simulink model "Dynamic_model_2021a"  (R2021a)
settings: Solver=VariableStepAuto  StartTime=0.0  StopTime=10.0  RelTol=1e-3
libraries: dspmtrx3 x1, sharedtransform x1
settings Model: Creator=volko  LastModifiedBy=volko

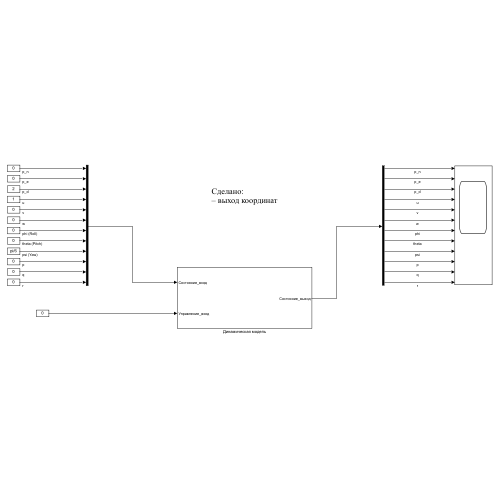
[thumbnail: Simulink's stored preview of the top-level diagram]
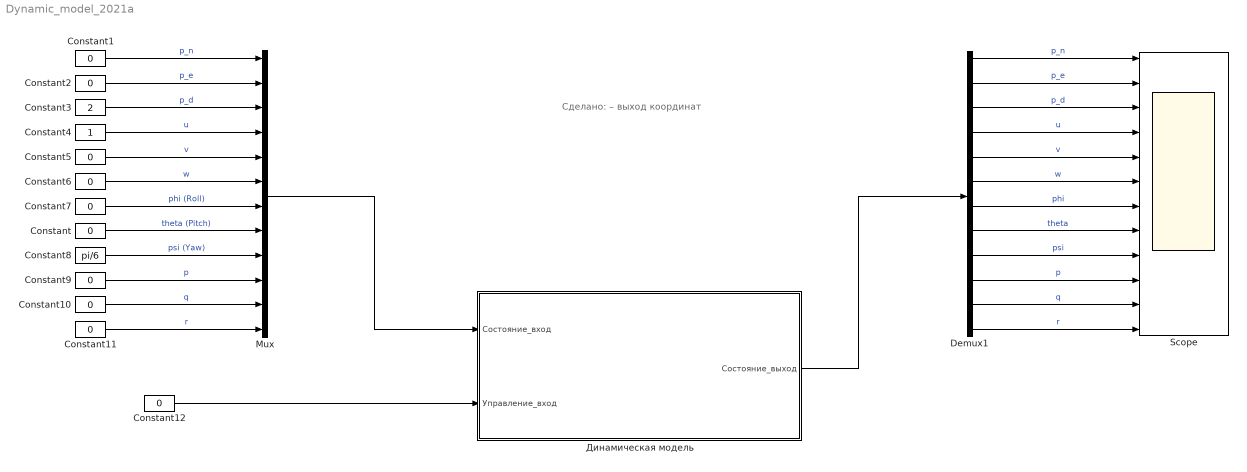
== system Dynamic_model_2021a ==
  note: Сделано:
      | – выход координат
  Constant{,1..2,5..7,9..12} (10 alike) : Constant  Value=0
  Constant3 : Constant  Value=2
  Constant4 : Constant
  Constant8 : Constant  Value=pi/6
  Demux1 : Demux  Outputs=12
  Mux : Mux  Inputs=12
  Scope : Scope  NumInputPorts=12
  Динамическая модель : Subsystem
  wires:
  Constant/1 -> Mux/8  "theta (Pitch)"
  Constant1/1 -> Mux/1  "p_n"
  Constant2/1 -> Mux/2  "p_e"
  Constant3/1 -> Mux/3  "p_d"
  Constant6/1 -> Mux/6  "w"
  Constant5/1 -> Mux/5  "v"
  Constant7/1 -> Mux/7  "phi (Roll)"
  Constant9/1 -> Mux/10  "p"
  Constant8/1 -> Mux/9  "psi (Yaw)"
  Constant10/1 -> Mux/11  "q"
  Constant11/1 -> Mux/12  "r"
  Mux/1 -> Динамическая модель/1(Состояние_вход)
  Constant12/1 -> Динамическая модель/2(Управление_вход)
  Динамическая модель/1(Состояние_выход) -> Demux1/1
  Demux1/1 -> Scope/1  "p_n"
  Demux1/2 -> Scope/2  "p_e"
  Demux1/3 -> Scope/3  "p_d"
  Constant4/1 -> Mux/4  "u"
  Demux1/4 -> Scope/4  "u"
  Demux1/5 -> Scope/5  "v"
  Demux1/6 -> Scope/6  "w"
  Demux1/7 -> Scope/7  "phi"
  Demux1/8 -> Scope/8  "theta"
  Demux1/9 -> Scope/9  "psi"
  Demux1/10 -> Scope/10  "p"
  Demux1/11 -> Scope/11  "q"
  Demux1/12 -> Scope/12  "r"

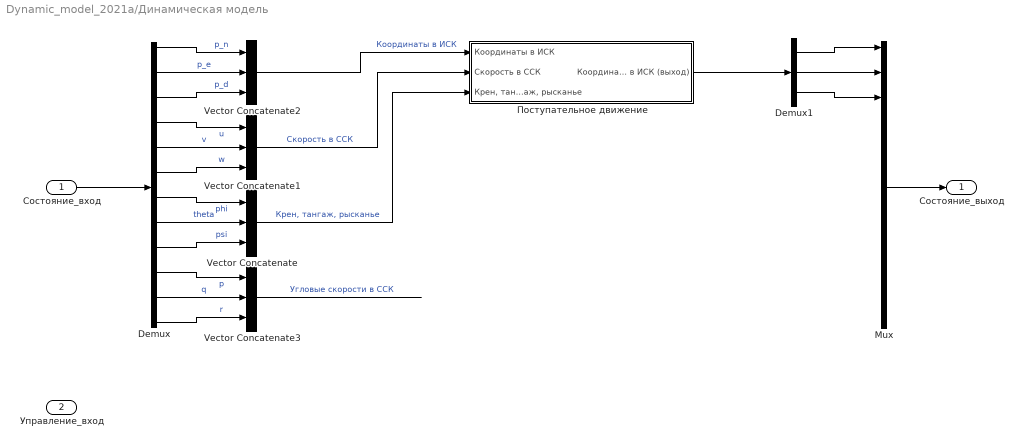
== system Dynamic_model_2021a/Динамическая модель ==
  Состояние_вход : Inport
  Управление_вход : Inport  Port=2
  Demux : Demux  Outputs=12
  Demux1 : Demux  Outputs=3
  Mux : Mux  Inputs=12
  Vector Concatenate{,1..3} (4 alike) : Concatenate  NumInputs=3
  Поступательное движение : Subsystem
  Состояние_выход : Outport
  wires:
  Состояние_вход/1 -> Demux/1
  Demux/1 -> Vector Concatenate2/1  "p_n"
  Demux/2 -> Vector Concatenate2/2  "p_e"
  Demux/3 -> Vector Concatenate2/3  "p_d"
  Demux/4 -> Vector Concatenate1/1  "u"
  Demux/5 -> Vector Concatenate1/2  "v"
  Demux/6 -> Vector Concatenate1/3  "w"
  Demux/7 -> Vector Concatenate/1  "phi"
  Demux/8 -> Vector Concatenate/2  "theta"
  Demux/9 -> Vector Concatenate/3  "psi"
  Demux/10 -> Vector Concatenate3/1  "p"
  Demux/11 -> Vector Concatenate3/2  "q"
  Demux/12 -> Vector Concatenate3/3  "r"
  Vector Concatenate2/1 -> Поступательное движение/1(Координаты в ИСК)  "Координаты в ИСК"
  Vector Concatenate1/1 -> Поступательное движение/2(Скорость в ССК)  "Скорость в ССК"
  Vector Concatenate/1 -> Поступательное движение/3("Крен, тангаж, рысканье")  "Крен, тангаж, рысканье"
  Поступательное движение/1(Координаты в ИСК (выход)) -> Demux1/1
  Vector Concatenate3/1 -> ?  "Угловые скорости в ССК"
  Mux/1 -> Состояние_выход/1
  Demux1/1 -> Mux/1
  Demux1/2 -> Mux/2
  Demux1/3 -> Mux/3

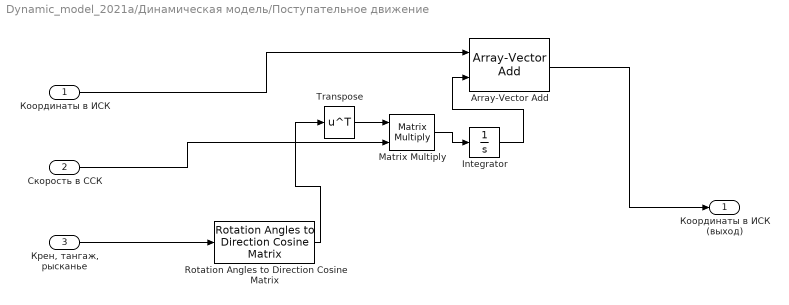
== system Dynamic_model_2021a/Динамическая модель/Поступательное движение ==
  Координаты в ИСК : Inport
  Скорость в ССК : Inport  Port=2
  "Крен, тангаж, рысканье" : Inport  Port=3
  Array-Vector Add : dspmtrx3/Array-Vector Add  Dimension=1  V_Source=Input port  V_VectFromMask=[0.5 0.25]  prodOutputSignedness=Auto  roundingMode=Floor  overflowMode=off  firstCoeffSignedness=Auto  firstCoeffDataTypeStr=Inherit: Same word length as input  firstCoeffMin=[]  firstCoeffMax=[]  firstCoeffLastDataTypeStr=Inherit: Same word length as input  accumSignedness=Auto  outputSignedness=Auto  outputDataTypeStr=Inherit: Same as accumulator  outputMin=[]  outputMax=[]  outputLastDataTypeStr=Inherit: Same as accumulator
      settings: SourceProductBaseCode=DS
  Integrator : Integrator
  Matrix Multiply : Product  Multiplication=Matrix(*)
  Rotation Angles to Direction Cosine Matrix : sharedtransform/Rotation Angles to Direction Cosine Matrix  rotationOrder=XYZ  aMode=aMode
      settings: SourceProductBaseCode=AE,PW,DR,MT,UV,VE
  Transpose : Math  Operator=transpose  SaturateOnIntegerOverflow=on
  Координаты в ИСК (выход) : Outport
  wires:
  Скорость в ССК/1 -> Matrix Multiply/2
  Integrator/1 -> Array-Vector Add/2
  Rotation Angles to Direction Cosine Matrix/1 -> Transpose/1
  Transpose/1 -> Matrix Multiply/1
  "Крен, тангаж, рысканье"/1 -> Rotation Angles to Direction Cosine Matrix/1
  Array-Vector Add/1 -> Координаты в ИСК (выход)/1
  Координаты в ИСК/1 -> Array-Vector Add/1
  Matrix Multiply/1 -> Integrator/1
